simulink model "Robot_Sim_bkp"  (R2017a)
settings: Solver=VariableStepAuto  StartTime=0.0  StopTime=Tsim  FixedStep=Ts_compute  RelTol=1e-3
values from neighbouring files (symbols this model uses):
  A = [0 ur2 0;-ur2 0 ur1;0 0 0]    [Model_old.m]    (also in PIController.m)
  b = 0.1    [Model_old.m]
  C = eye(3)    [Model_old.m]    (also in PIController.m)
  g = 40    [Model_old.m]    (also in ModeloBase_OLD.m)
  Gyro_bias = 0.004    [Model_old.m]
  Kd = 0    [Model_old.m]
  Ki = 10.0    (= 10)    [Model_old.m]
  Kp = 5.0    (= 5)    [Model_old.m]
  ksi = 0.6    [Model_old.m]    (also in ModeloBase_OLD.m = 0.3)
  Rv = var(noise.data)    [Model_old.m]
  Ts = 0.1    [Model_old.m]    (also in ModeloBase_OLD.m; PIController.m)
  Ts_sensor = 1/50    (= 0.02)    [Model_old.m]
undefined symbols (not defined in the file or in its folder): DiscIntNeverNeededParam, K_LQ, Rn, Rw, Ts_compute, Vd
libraries: simulink x27, cstblocks x11
settings Model: PauseTimes=28  NumberOfSteps=10  Creator=davi2  LastModifiedBy=marcus

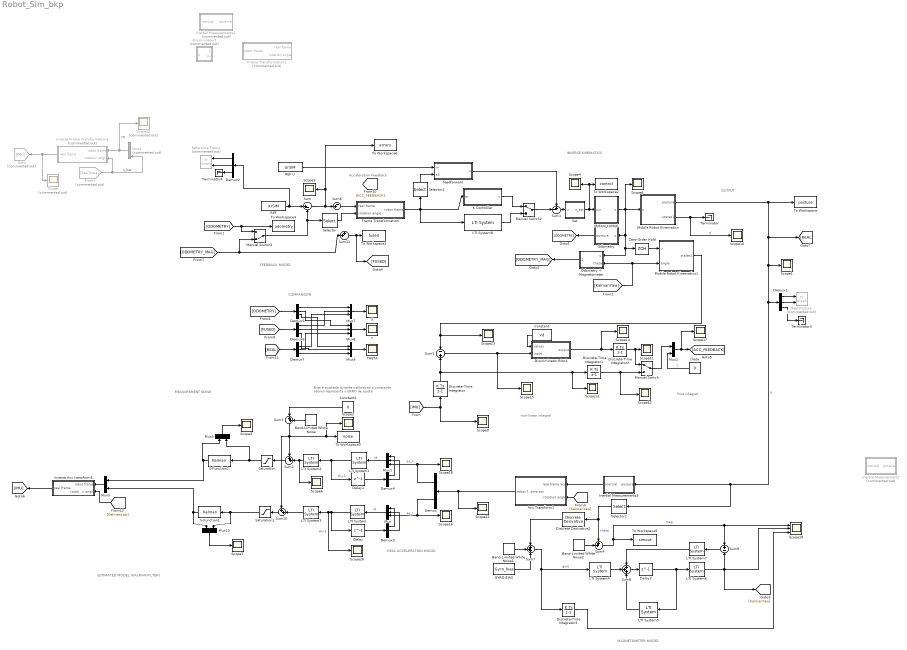
== system Robot_Sim_bkp ==
  note: COMPARISON
  note: Bias é ajustada durante calibracao
      | a constante abaixo representa o ERRO de ajuste
  note: Pure integral
  note: Acceleration Feedback
  note: OUTPUT
  note: MEASUREMENT NOISE
  note: REAL ACCELERATION
      | MODEL
  note: INVERSE KINEMATICS
  note: MAGNETOMETER MODEL
  note: FEEDBACK MODEL
  note: ESTIMATED MODEL (KALMAN FILTER)
  note: non-linear integral
  Acc Transform1 : Subsystem
  Band-Limited White Noise : simulink/Sources/Band-Limited White Noise  Cov=0.0001  Ts=Ts_sensor  seed=[23341]
  Band-Limited White Noise1 : simulink/Sources/Band-Limited White Noise  Cov=0.00001  Ts=Ts_sensor  seed=[23341]
  Band-Limited White Noise2 : simulink/Sources/Band-Limited White Noise  Cov=Rn^2  Ts=Ts_sensor  seed=[23341]
  Constant : Constant  Value=Vd
  Constant2 : Constant  Value=0
  Delay : Delay  DelayLength=1
  Delay1 : Delay  DelayLength=1
  Delay2 : Delay  DelayLength=1
  Demux : Demux  Outputs=2
  Demux{1..7} (7 alike) : Demux  Outputs=3
  Discrete Derivative2 : simulink/Discrete/Discrete Derivative  gainval=1.0  ICPrevScaledInput=0.0  OutMin=[]  OutMax=[]  OutDataType=fixdt(1, 16)  OutScaling=2^-10  DoSatur=off
  Discrete-Time Integrator : DiscreteIntegrator  InitialConditionSetting=State (most efficient)  SampleTime=-1  ICPrevOutput=DiscIntNeverNeededParam  ICPrevScaledInput=DiscIntNeverNeededParam
  Discrete-Time Integrator1 : DiscreteIntegrator  InitialConditionSetting=State (most efficient)  SampleTime=Ts_sensor  ICPrevOutput=DiscIntNeverNeededParam  ICPrevScaledInput=DiscIntNeverNeededParam
  Discrete-Time Integrator2 : DiscreteIntegrator  InitialConditionSetting=State (most efficient)  SampleTime=Ts_sensor  ICPrevOutput=DiscIntNeverNeededParam  ICPrevScaledInput=DiscIntNeverNeededParam
  Discrete-Time Integrator3 : DiscreteIntegrator  InitialConditionSetting=State (most efficient)  SampleTime=-1  ICPrevOutput=DiscIntNeverNeededParam  ICPrevScaledInput=DiscIntNeverNeededParam
  Discriminator Block : Subsystem
  Frame Transformation : Subsystem
  Frame Transformation1 : Subsystem  Commented=on
  From5 : From  Commented=on  GotoTag=RealTheta
  GYRO BIAS : Constant  Value=Gyro_bias
  Goto : Goto  Commented=on  GotoTag=IMU
  Inertial Measurements : Subsystem  Commented=on
  Inertial Measurements1 : Subsystem  Commented=on
  Inertial Measurements3 : Subsystem
  Inverse Acc transform1 : Subsystem
  Inverse Frame Transformation1 : Subsystem  Commented=on
  K Controller : Subsystem
  LTI System : cstblocks/LTI System  sys=A  IC=[]
  LTI System1 : cstblocks/LTI System  sys=A  IC=[]
  LTI System2 : cstblocks/LTI System  sys=C  IC=[]
  LTI System3 : cstblocks/LTI System  sys=C  IC=[]
  LTI System4 : cstblocks/LTI System  sys=Bs  IC=[]
  LTI System5 : cstblocks/LTI System  sys=As  IC=[]
  LTI System6 : cstblocks/LTI System  sys=Cs  IC=[]
  LTI System7 : cstblocks/LTI System  sys=K_KALM  IC=[]
  LTI System8 : cstblocks/LTI System  sys=-K_LQ  IC=[]
  Manual Switch : ManualSwitch
  Manual Switch1 : ManualSwitch  CurrentSetting=0
  Manual Switch2 : ManualSwitch
  Mobile Robot Kinematics : Subsystem
  Mobile Robot Kinematics1 : Subsystem
  Motors control : Subsystem
  Mux{,1,7..9} (5 alike) : Mux  Inputs=3
  Mux{2..3,5,10} (4 alike) : Mux  Inputs=2
  Mux4 : Mux  Commented=on  Inputs=3
  Odometry : Subsystem
  Odometry + Magnetometer : Subsystem
  REF : FromWorkspace  VariableName=XrSIM  SampleTime=Ts  OutputAfterFinalValue=Holding final value
  REF U : FromWorkspace  VariableName=UrSIM  SampleTime=Ts  OutputAfterFinalValue=Holding final value
  Real Posture : simulink/Sinks/XY Graph  Commented=on  xmin=0  xmax=3  ymin=-0.8  ymax=1.5  st=Ts
  Reference Frame : simulink/Sinks/XY Graph  Commented=on  xmin=0  xmax=2  ymin=0  ymax=1.5  st=Ts
  S-Function1 : S-Function  FunctionName=Kalman  Parameters=Ts_sensor,A,C,Rw,Rv  SFunctionDeploymentMode=off  EnableBusSupport=off  mask{Ts=Ts_sensor, A=A, C=C, Rv=Rv, Rw=Rw}
      mask prompts: Ts "Tempo de Amostragem"; A "Matriz A"; C "Matriz C"; Rv "Covariancia da Saida"; Rw "Covariancia do Processo"
      mask DialogControl DescTextVar Tooltip: Filtro
      mask Display: disp('MyKalman')
  S-Function2 : S-Function  FunctionName=Kalman  Parameters=Ts_sensor,A,C,Rw,Rv  SFunctionDeploymentMode=off  EnableBusSupport=off  mask{Ts=Ts_sensor, A=A, C=C, Rv=Rv, Rw=Rw}
      mask prompts: Ts "Tempo de Amostragem"; A "Matriz A"; C "Matriz C"; Rv "Covariancia da Saida"; Rw "Covariancia do Processo"
      mask DialogControl DescTextVar Tooltip: Filtro
      mask Display: disp('MyKalman')
  Sat : Subsystem
  Saturation : Saturate  UpperLimit=4*9.8  LowerLimit=-4*9.8
  Saturation1 : Saturate  UpperLimit=4*9.8  LowerLimit=-4*9.8
  Scope : Scope  Commented=on
  Scope{1..18,22..23,26} (21 alike) : Scope
  Scope19 : Scope  NumInputPorts=3
  Scope21 : Scope  Commented=on
  Selector : Selector  InputPortWidth=3  IndexOptions=Index vector (dialog)  Indices=3  OutputSizes=1
  Selector1 : Selector  InputPortWidth=3  IndexOptions=Index vector (dialog)  Indices=3  OutputSizes=1
  Selector2 : Selector  InputPortWidth=3  IndexOptions=Index vector (dialog)  Indices=3  OutputSizes=1
  Sum : Sum  Inputs=|+-
  Sum1 : Sum  Inputs=+-|
  Sum{2,4,10..11} (4 alike) : Sum  Inputs=++|
  Sum3 : Sum  Inputs=|++
  Sum5 : Sum  Inputs=-+
  Sum6 : Sum  Inputs=-+|
  Sum7 : Sum  Inputs=+++
  Sum8 : Sum  Inputs=+++
  Sum9 : Sum  Inputs=+-
  THETA : Scope
  Terminator : Terminator
  Terminator3 : Terminator
  Terminator4 : Terminator
  To Workspace : ToWorkspace  VariableName=posture  SaveFormat=Timeseries  SampleTime=-1
  To Workspace1 : ToWorkspace  VariableName=fused  SaveFormat=Timeseries  SampleTime=-1
  To Workspace2 : ToWorkspace  VariableName=control  SaveFormat=Timeseries  SampleTime=-1
  To Workspace3 : ToWorkspace  VariableName=noise  SaveFormat=Timeseries  SampleTime=-1
  To Workspace4 : ToWorkspace  VariableName=odometry  SaveFormat=Timeseries  SampleTime=-1
  To Workspace5 : ToWorkspace  VariableName=simout  SaveFormat=Timeseries  SampleTime=-1
  To Workspace6 : ToWorkspace  VariableName=errors  SaveFormat=Timeseries  SampleTime=-1
  X : Scope
  Y : Scope
  Zero-Order Hold : ZeroOrderHold  SampleTime=-1
  discriminator5 : Subsystem  Commented=on
  feedforward : Subsystem
  theta : Constant  Value=0
  wires:
  Frame Transformation/1(robot frame) -> LTI System8/1, K Controller/1(er), Selector1/1
  REF U/1 -> feedforward/1(ur)
  Selector1/1 -> feedforward/2(e3)
  Motors control/1(u) -> Odometry + Magnetometer/1(u), Zero-Order Hold/1, Odometry/1(u), Mobile Robot Kinematics/1(u), Scope8/1
  Selector2/1 -> Sum4/1, Discrete Derivative2/1  "theta"
  Demux1/1 -> Real Posture/1
  Demux1/2 -> Real Posture/2
  REF/1 -> Demux2/1, Sum/1
  Odometry/1(posture) -> [ODOMETRY]
  Sum1/1 -> Sat/1(u)
  Sat/1(u_sat) -> Motors control/1(uin), Scope4/1, To Workspace2/1
  Demux1/3 -> Terminator3/1
  Band-Limited White Noise2/1 -> Sum4/2
  Demux2/1 -> Reference Frame/1
  Demux2/2 -> Reference Frame/2
  Demux2/3 -> Terminator4/1
  LTI System/1 -> Scope26/1, LTI System3/1, Delay/1  "xk+1"
  Delay/1 -> Demux3/1
  Demux3/1 -> Mux/1
  Demux3/2 -> Mux/2
  Mux/1 -> LTI System/1  "xk"
  Demux4/2 -> Mux1/2
  Delay1/1 -> Demux4/1
  Demux4/1 -> Mux1/1
  LTI System1/1 -> Delay1/1, LTI System2/1  "xk+1"
  Mux1/1 -> LTI System1/1  "xk"
  Inverse Frame Transformation1/1(real frame) -> Goto/1, Scope/1
  From5/1 -> Mux4/3, Inverse Frame Transformation1/2(rotation angle)  "t_hat"
  LTI System3/1 -> Sum10/2
  Mux4/1 -> Scope21/1, Inverse Frame Transformation1/1(robot frame)  "im"
  Mobile Robot Kinematics/1(posture) -> [REAL], Selector2/1, Inertial Measurements3/1(posture), Demux1/1, Scope1/1, To Workspace/1  "P"
  Demux/1 -> Mux1/3, Scope18/1  "ax_r"
  Demux/2 -> Scope16/1, Mux/3  "ay_r"
  Inertial Measurements3/1(inercial) -> Acc Transform1/1(real frame acc)
  Acc Transform1/1(robot frame acc) -> Scope22/1, Demux/1
  Sum6/1 -> Frame Transformation/1(real frame)
  theta/1 -> Mux2/2  "t"
  Mux2/1 -> Scope17/1, [ACC_FEEDBACK]
  LTI System2/1 -> Scope6/1, Sum2/2
  Sum11/1 -> [FUSED], To Workspace1/1
  Mux5/1 -> Scope5/1
  Discrete-Time Integrator2/1 -> Scope11/1, Manual Switch/1
  Discrete-Time Integrator1/1 -> Manual Switch/2, Scope12/1
  Manual Switch/1 -> Mux2/1
  Discriminator Block/1(output) -> Discrete-Time Integrator2/1, Scope14/1
  Selector/1 -> Frame Transformation/2(rotation angle)
  [KalmanYaw] -> Acc Transform1/2(rotation angle)
  Odometry + Magnetometer/1(posture) -> [ODOMETRY_MAG]
  [KalmanYaw] -> Odometry + Magnetometer/2(theta), Mobile Robot Kinematics1/2(angle)
  [ODOMETRY] -> Manual Switch1/1, To Workspace4/1
  [ODOMETRY_MAG] -> Sum11/2, Manual Switch1/2
  Manual Switch1/1 -> Selector/1, Sum/2
  [ODOMETRY] -> Demux5/1
  [FUSED] -> Demux6/1
  [REAL] -> Demux7/1
  Demux5/1 -> Mux7/1
  Demux6/1 -> Mux7/2
  Demux7/1 -> Mux7/3
  Mux7/1 -> X/1
  Demux5/2 -> Mux8/1
  Demux6/2 -> Mux8/2
  Demux7/2 -> Mux8/3
  Demux5/3 -> Mux9/1
  Demux6/3 -> Mux9/2
  Demux7/3 -> Mux9/3
  Mux8/1 -> Y/1
  Mux9/1 -> THETA/1
  Mobile Robot Kinematics/2(states1) -> Scope10/1, Terminator/1  "p'"
  Mux3/1 -> Inverse Acc transform1/1(robot frame)
  [KalmanYaw] -> Inverse Acc transform1/2(rotation angle)
  Inverse Acc transform1/1(real frame) -> [IMU]
  Constant/1 -> Discriminator Block/1(values)
  Sum3/1 -> Sum10/1, Sum2/1, Scope2/1, To Workspace3/1
  Band-Limited White Noise/1 -> Sum3/2
  Constant2/1 -> Sum3/1
  Sum10/1 -> Saturation1/1
  Sum2/1 -> Saturation/1
  Saturation1/1 -> S-Function1/1, Mux10/2
  Saturation/1 -> S-Function2/1, Mux5/2
  Mux10/1 -> Scope7/1
  Zero-Order Hold/1 -> Mobile Robot Kinematics1/1(u)
  [IMU] -> Discrete-Time Integrator/1, Scope9/1
  Sum5/1 -> Scope15/1, Discriminator Block/2(input)
  Discrete-Time Integrator/1 -> Scope13/1, Discrete-Time Integrator1/1, Sum5/2
  S-Function1/1 -> Mux3/2, Mux10/1
  Mobile Robot Kinematics1/1(states1) -> Scope23/1, Sum5/1
  S-Function2/1 -> Mux3/1, Mux5/1
  Band-Limited White Noise1/1 -> Sum7/2
  Discrete Derivative2/1 -> Sum7/1
  GYRO BIAS/1 -> Sum7/3
  Sum7/1 -> Discrete-Time Integrator3/1, LTI System4/1  "gyro"
  Sum4/1 -> To Workspace5/1, Scope19/1, Sum9/1  "mag"
  Sum8/1 -> Delay2/1
  LTI System4/1 -> Sum8/2
  Delay2/1 -> LTI System6/1, LTI System5/1
  LTI System5/1 -> Sum8/3
  LTI System7/1 -> Sum8/1
  LTI System6/1 -> Scope19/2, [KalmanYaw], Sum9/2
  Sum9/1 -> LTI System7/1
  Discrete-Time Integrator3/1 -> Scope19/3
  Sum/1 -> Sum6/2, To Workspace6/1, Scope3/1
  Manual Switch2/1 -> Sum1/2
  feedforward/1(u) -> Sum1/1
  LTI System8/1 -> Manual Switch2/2
  K Controller/1(v) -> Manual Switch2/1

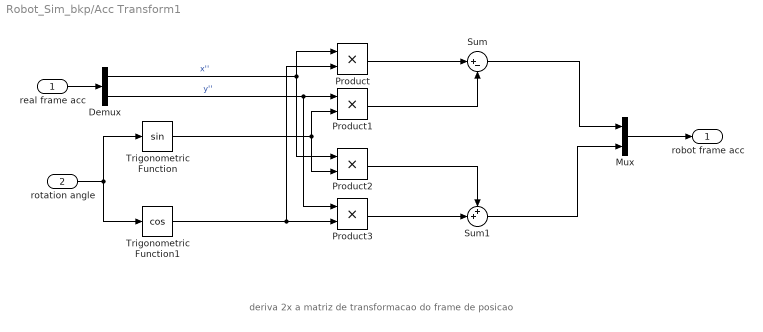
== system Robot_Sim_bkp/Acc Transform1 ==
  note: deriva 2x a matriz de transformacao do frame de posicao
  real frame acc : Inport
  rotation angle : Inport  Port=2
  Demux : Demux  Outputs=2
  Mux : Mux  Inputs=2
  Product{,1..3} (4 alike) : Product
  Sum : Sum  Inputs=|+-
  Sum1 : Sum  Inputs=++|
  Trigonometric Function : Trigonometry
  Trigonometric Function1 : Trigonometry  Operator=cos
  robot frame acc : Outport
  wires:
  rotation angle/1 -> Trigonometric Function/1, Trigonometric Function1/1
  Mux/1 -> robot frame acc/1
  real frame acc/1 -> Demux/1
  Demux/1 -> Product2/1, Product/1  "x''"
  Trigonometric Function1/1 -> Product/2, Product3/2
  Product/1 -> Sum/1
  Trigonometric Function/1 -> Product1/2, Product2/2
  Demux/2 -> Product3/1, Product1/1  "y''"
  Product1/1 -> Sum/2
  Sum/1 -> Mux/1
  Product3/1 -> Sum1/2
  Product2/1 -> Sum1/1
  Sum1/1 -> Mux/2

== system Robot_Sim_bkp/Discriminator Block ==
  values : Inport
  input : Inport  Port=2
  Demux : Demux  Outputs=2
  Mux : Mux  Inputs=2
  discriminator1 : Subsystem
  discriminator3 : Subsystem
  output : Outport
  wires:
  input/1 -> Demux/1
  Demux/1 -> discriminator3/2(IN)
  Demux/2 -> discriminator1/2(IN)
  Mux/1 -> output/1
  discriminator3/1(OUT) -> Mux/1
  discriminator1/1(OUT) -> Mux/2
  values/1 -> discriminator1/1(value), discriminator3/1(value)

== system Robot_Sim_bkp/Frame Transformation ==
  real frame : Inport
  rotation angle : Inport  Port=2
  Mux : Mux  Inputs=2
  S-Function : S-Function  FunctionName=Real2Robot  Parameters=Ts  SFunctionDeploymentMode=off  EnableBusSupport=off
  robot frame : Outport
  wires:
  real frame/1 -> Mux/1
  rotation angle/1 -> Mux/2
  Mux/1 -> S-Function/1
  S-Function/1 -> robot frame/1

== system Robot_Sim_bkp/Frame Transformation1 ==
  real frame : Inport
  rotation angle : Inport  Port=2
  Mux : Mux  Inputs=2
  S-Function : S-Function  FunctionName=Real2Robot  Parameters=Ts_compute  SFunctionDeploymentMode=off  EnableBusSupport=off
  robot frame : Outport
  wires:
  real frame/1 -> Mux/1
  rotation angle/1 -> Mux/2
  Mux/1 -> S-Function/1
  S-Function/1 -> robot frame/1

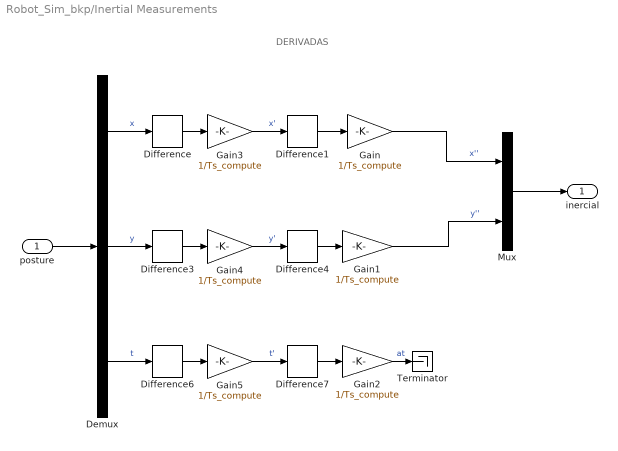
== system Robot_Sim_bkp/Inertial Measurements ==
  note: DERIVADAS
  posture : Inport
  Demux : Demux  Outputs=3
  Difference{,1,3..4,6..7} (6 alike) : simulink/Discrete/Difference  ICPrevInput=0.0  OutMin=[]  OutMax=[]  OutDataType=fixdt(1, 16)  OutScaling=2^-10  DoSatur=off
  Gain{,1..5} (6 alike) : Gain  Gain=1/Ts_compute
  Mux : Mux  Inputs=2
  Terminator : Terminator
  inercial : Outport
  wires:
  posture/1 -> Demux/1
  Demux/3 -> Difference6/1  "t"
  Demux/2 -> Difference3/1  "y"
  Demux/1 -> Difference/1  "x"
  Difference1/1 -> Gain/1
  Difference4/1 -> Gain1/1
  Difference7/1 -> Gain2/1
  Mux/1 -> inercial/1
  Gain2/1 -> Terminator/1  "at"
  Difference/1 -> Gain3/1
  Gain3/1 -> Difference1/1  "x'"
  Difference3/1 -> Gain4/1
  Gain4/1 -> Difference4/1  "y'"
  Difference6/1 -> Gain5/1
  Gain5/1 -> Difference7/1  "t'"
  Gain/1 -> Mux/1  "x''"
  Gain1/1 -> Mux/2  "y''"

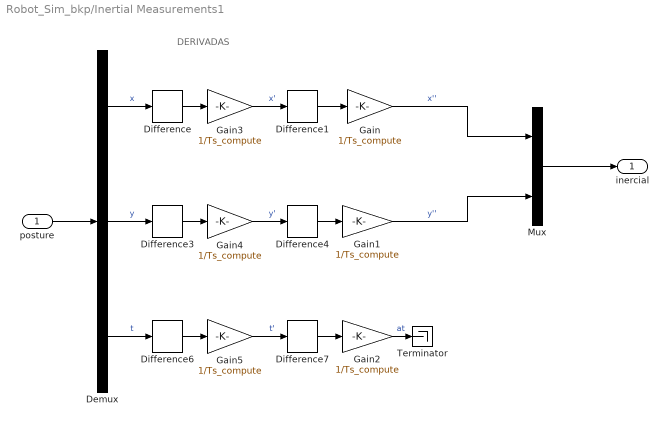
== system Robot_Sim_bkp/Inertial Measurements1 ==
  note: DERIVADAS
  posture : Inport
  Demux : Demux  Outputs=3
  Difference{,1,3..4,6..7} (6 alike) : simulink/Discrete/Difference  ICPrevInput=0.0  OutMin=[]  OutMax=[]  OutDataType=fixdt(1, 16)  OutScaling=2^-10  DoSatur=off
  Gain{,1..5} (6 alike) : Gain  Gain=1/Ts_compute
  Mux : Mux  Inputs=2
  Terminator : Terminator
  inercial : Outport
  wires:
  posture/1 -> Demux/1
  Demux/3 -> Difference6/1  "t"
  Demux/2 -> Difference3/1  "y"
  Demux/1 -> Difference/1  "x"
  Difference1/1 -> Gain/1
  Difference4/1 -> Gain1/1
  Difference7/1 -> Gain2/1
  Mux/1 -> inercial/1
  Gain2/1 -> Terminator/1  "at"
  Difference/1 -> Gain3/1
  Gain3/1 -> Difference1/1  "x'"
  Difference3/1 -> Gain4/1
  Gain4/1 -> Difference4/1  "y'"
  Difference6/1 -> Gain5/1
  Gain5/1 -> Difference7/1  "t'"
  Gain/1 -> Mux/1  "x''"
  Gain1/1 -> Mux/2  "y''"

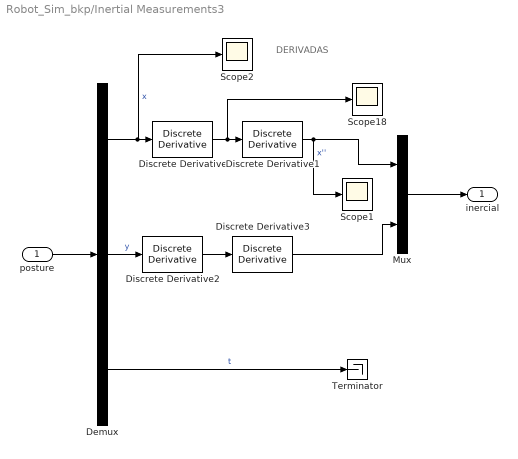
== system Robot_Sim_bkp/Inertial Measurements3 ==
  note: DERIVADAS
  posture : Inport
  Demux : Demux  Outputs=3
  Discrete Derivative{,1..3} (4 alike) : simulink/Discrete/Discrete Derivative  gainval=1.0  ICPrevScaledInput=0.0  OutMin=[]  OutMax=[]  OutDataType=fixdt(1, 16)  OutScaling=2^-10  DoSatur=off
  Mux : Mux  Inputs=2
  Scope1 : Scope
  Scope18 : Scope
  Scope2 : Scope
  Terminator : Terminator
  inercial : Outport
  wires:
  posture/1 -> Demux/1
  Demux/1 -> Discrete Derivative/1, Scope2/1  "x"
  Mux/1 -> inercial/1
  Discrete Derivative1/1 -> Scope1/1, Mux/1  "x''"
  Discrete Derivative/1 -> Scope18/1, Discrete Derivative1/1
  Demux/2 -> Discrete Derivative2/1  "y"
  Discrete Derivative2/1 -> Discrete Derivative3/1
  Discrete Derivative3/1 -> Mux/2
  Demux/3 -> Terminator/1  "t"

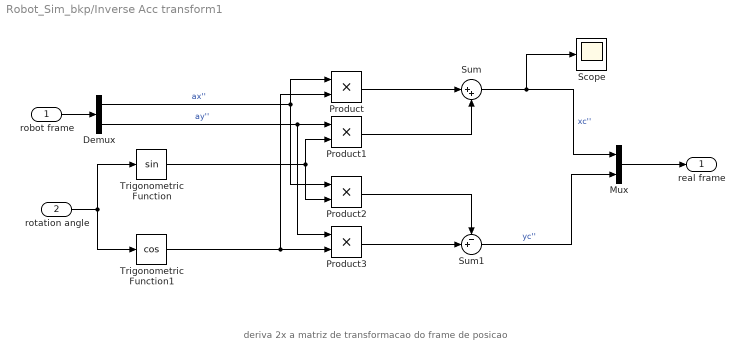
== system Robot_Sim_bkp/Inverse Acc transform1 ==
  note: deriva 2x a matriz de transformacao do frame de posicao
  robot frame : Inport
  rotation angle : Inport  Port=2
  Demux : Demux  Outputs=2
  Mux : Mux  Inputs=2
  Product{,1..3} (4 alike) : Product
  Scope : Scope
  Sum : Sum  Inputs=|++
  Sum1 : Sum  Inputs=-+|
  Trigonometric Function : Trigonometry
  Trigonometric Function1 : Trigonometry  Operator=cos
  real frame : Outport
  wires:
  rotation angle/1 -> Trigonometric Function/1, Trigonometric Function1/1
  Mux/1 -> real frame/1
  robot frame/1 -> Demux/1
  Demux/1 -> Product2/1, Product/1  "ax''"
  Trigonometric Function1/1 -> Product/2, Product3/2
  Product/1 -> Sum/1
  Trigonometric Function/1 -> Product1/2, Product2/2
  Demux/2 -> Product3/1, Product1/1  "ay''"
  Product1/1 -> Sum/2
  Sum/1 -> Scope/1, Mux/1  "xc''"
  Product3/1 -> Sum1/2
  Product2/1 -> Sum1/1
  Sum1/1 -> Mux/2  "yc''"

== system Robot_Sim_bkp/Inverse Frame Transformation1 ==
  robot frame : Inport
  rotation angle : Inport  Port=2
  Mux : Mux  Inputs=2
  S-Function : S-Function  FunctionName=Robot2Real  Parameters=Ts  SFunctionDeploymentMode=off  EnableBusSupport=off
  real frame : Outport
  wires:
  S-Function/1 -> real frame/1
  Mux/1 -> S-Function/1
  rotation angle/1 -> Mux/2
  robot frame/1 -> Mux/1

== system Robot_Sim_bkp/K Controller ==
  er : Inport
  Constant : Constant  Value=ksi
  Constant1 : Constant  Value=g
  Mux : Mux  Inputs=5
  S-Function : S-Function  FunctionName=ControllerK  Parameters=Ts  SFunctionDeploymentMode=off  EnableBusSupport=off
  v : Outport
  wires:
  er/1 -> Mux/1
  [vr] -> Mux/2
  [wr] -> Mux/3
  Constant/1 -> Mux/4
  Constant1/1 -> Mux/5
  Mux/1 -> S-Function/1
  S-Function/1 -> v/1

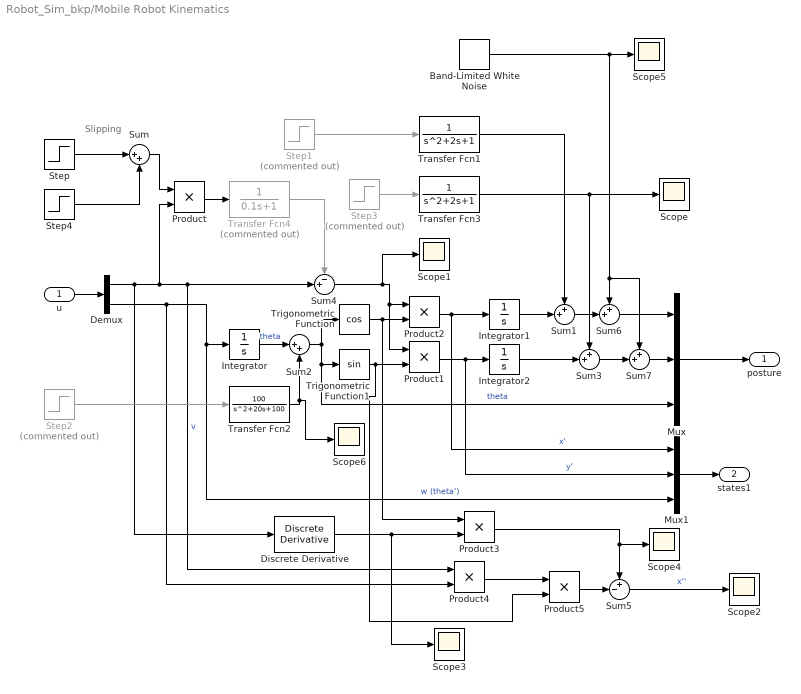
== system Robot_Sim_bkp/Mobile Robot Kinematics ==
  note: Slipping
  u : Inport
  Band-Limited White Noise : simulink/Sources/Band-Limited White Noise  Cov=0  Ts=0.05  seed=[23341]
  Demux : Demux  Outputs=2
  Discrete Derivative : simulink/Discrete/Discrete Derivative  gainval=1.0  ICPrevScaledInput=0.0  OutMin=[]  OutMax=[]  OutDataType=fixdt(1, 16)  OutScaling=2^-10  DoSatur=off
  Integrator : Integrator
  Integrator1 : Integrator
  Integrator2 : Integrator
  Mux : Mux  Inputs=3
  Mux1 : Mux  Inputs=3
  Product{,1..5} (6 alike) : Product
  Scope{,1..6} (7 alike) : Scope
  Step : Step  Time=25  SampleTime=0
  Step1 : Step  Commented=on  Time=20  After=0.7  SampleTime=0
  Step2 : Step  Commented=on  Time=10  After=0.5  SampleTime=0
  Step3 : Step  Commented=on  Time=5  After=-0.7  SampleTime=0
  Step4 : Step  Time=27  After=-1  SampleTime=0
  Sum : Sum  Inputs=|++
  Sum{1,3,6..7} (4 alike) : Sum  Inputs=++|
  Sum2 : Sum  Inputs=|++
  Sum4 : Sum  Inputs=-+|
  Sum5 : Sum  Inputs=+-|
  Transfer Fcn1 : TransferFcn  Numerator=1
  Transfer Fcn2 : TransferFcn  Numerator=100  Denominator=[1 20 100]
  Transfer Fcn3 : TransferFcn  Numerator=1
  Transfer Fcn4 : TransferFcn  Commented=on  Numerator=1  Denominator=[0.1 1]
  Trigonometric Function : Trigonometry  Operator=cos
  Trigonometric Function1 : Trigonometry
  posture : Outport
  states1 : Outport  Port=2
  wires:
  u/1 -> Demux/1
  Demux/2 -> Product4/2, Integrator/1, Mux1/3  "w (theta')"
  Trigonometric Function/1 -> Product3/1, Product2/2
  Demux/1 -> Discrete Derivative/1, Product4/1, Sum4/2, Product/2  "v"
  Trigonometric Function1/1 -> Product5/2, Product1/2
  Mux/1 -> posture/1
  Step2/1 -> Transfer Fcn2/1
  Integrator/1 -> Sum2/1  "theta"
  Sum2/1 -> Mux/3, Trigonometric Function1/1, Trigonometric Function/1  "theta"
  Transfer Fcn2/1 -> Scope6/1, Sum2/2
  Product1/1 -> Mux1/2, Integrator2/1  "y'"
  Product2/1 -> Mux1/1, Integrator1/1  "x'"
  Step1/1 -> Transfer Fcn1/1
  Step3/1 -> Transfer Fcn3/1
  Integrator1/1 -> Sum1/2
  Integrator2/1 -> Sum3/2
  Transfer Fcn3/1 -> Sum3/1, Scope/1
  Transfer Fcn1/1 -> Sum1/1
  Step/1 -> Sum/1
  Step4/1 -> Sum/2
  Sum/1 -> Product/1
  Sum4/1 -> Scope1/1, Product1/1, Product2/1
  Product/1 -> Transfer Fcn4/1
  Transfer Fcn4/1 -> Sum4/1
  Mux1/1 -> states1/1
  Discrete Derivative/1 -> Scope3/1, Product3/2
  Product3/1 -> Scope4/1, Sum5/1
  Sum5/1 -> Scope2/1  "x''"
  Product4/1 -> Product5/1
  Product5/1 -> Sum5/2
  Sum1/1 -> Sum6/2
  Sum3/1 -> Sum7/2
  Sum7/1 -> Mux/2
  Sum6/1 -> Mux/1
  Band-Limited White Noise/1 -> Scope5/1, Sum7/1, Sum6/1

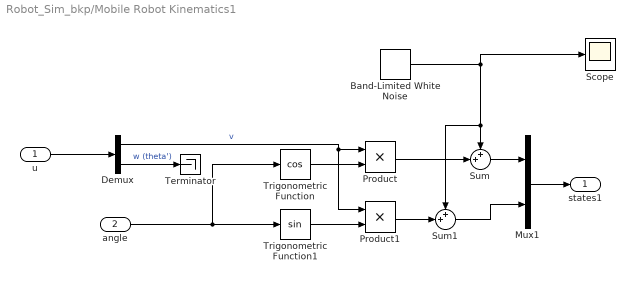
== system Robot_Sim_bkp/Mobile Robot Kinematics1 ==
  u : Inport
  angle : Inport  Port=2
  Band-Limited White Noise : simulink/Sources/Band-Limited White Noise  Cov=0.05^4  Ts=0.1  seed=[23341]
  Demux : Demux  Outputs=2
  Mux1 : Mux  Inputs=2
  Product : Product
  Product1 : Product
  Scope : Scope
  Sum : Sum  Inputs=++|
  Sum1 : Sum  Inputs=++|
  Terminator : Terminator
  Trigonometric Function : Trigonometry  Operator=cos
  Trigonometric Function1 : Trigonometry
  states1 : Outport
  wires:
  u/1 -> Demux/1
  Demux/1 -> Product1/1, Product/1  "v"
  Mux1/1 -> states1/1
  Trigonometric Function/1 -> Product/2
  Trigonometric Function1/1 -> Product1/2
  Product/1 -> Sum/2
  Product1/1 -> Sum1/2
  Band-Limited White Noise/1 -> Scope/1, Sum1/1, Sum/1
  Sum/1 -> Mux1/1
  Sum1/1 -> Mux1/2
  angle/1 -> Trigonometric Function/1, Trigonometric Function1/1
  Demux/2 -> Terminator/1  "w (theta')"

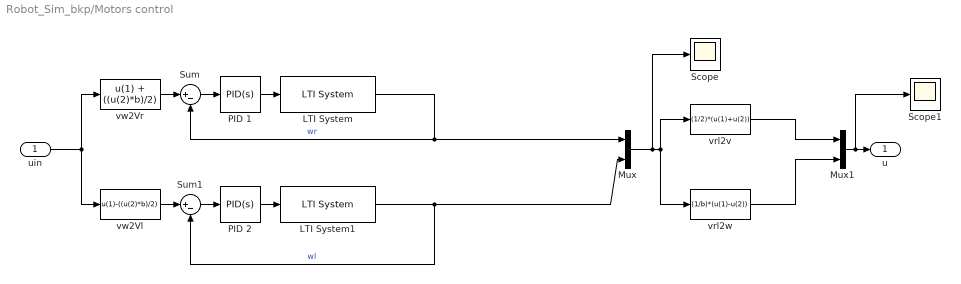
== system Robot_Sim_bkp/Motors control ==
  uin : Inport
  LTI System : cstblocks/LTI System  sys=HMotor  IC=[]
  LTI System1 : cstblocks/LTI System  sys=HMotor  IC=[]
  Mux : Mux  Inputs=2
  Mux1 : Mux  Inputs=2
  PID 1 : simulink/Continuous/PID Controller  Controller=PID  TimeDomain=Continuous-time  SampleTime=-1  IntegratorMethod=Forward Euler  FilterMethod=Forward Euler  Form=Parallel  UseFilter=on  ControllerParametersSource=internal  P=Kp  I=Ki  D=Kd  N=100  InitialConditionSource=internal  InitialConditionForIntegrator=0  InitialConditionForFilter=0  ExternalReset=none  LimitOutput=off  UpperSaturationLimit=inf  LowerSaturationLimit=-inf  LinearizeAsGain=on  AntiWindupMode=none  Kb=1  TrackingMode=off  Kt=1  PParamMin=[]  PParamMax=[]  IParamMin=[]  IParamMax=[]  DParamMin=[]  DParamMax=[]  NParamMin=[]  NParamMax=[]  KbParamMin=[]  KbParamMax=[]  KtParamMin=[]  KtParamMax=[]  POutMin=[]  POutMax=[]  IOutMin=[]  IOutMax=[]  DOutMin=[]  DOutMax=[]  NOutMin=[]  NOutMax=[]  KbOutMin=[]  KbOutMax=[]  KtOutMin=[]  KtOutMax=[]  IntegratorOutMin=[]  IntegratorOutMax=[]  FilterOutMin=[]  FilterOutMax=[]  SumOutMin=[]  SumOutMax=[]  SumI1OutMin=[]  SumI1OutMax=[]  SumI2OutMin=[]  SumI2OutMax=[]  SumI3OutMin=[]  SumI3OutMax=[]  SumDOutMin=[]  SumDOutMax=[]  SaturationOutMin=[]  SaturationOutMax=[]  IntegratorContinuousStateAttributes=''  IntegratorStateMustResolveToSignalObject=off  IntegratorRTWStateStorageClass=Auto  FilterContinuousStateAttributes=''  FilterStateMustResolveToSignalObject=off  FilterRTWStateStorageClass=Auto  DifferentiatorICPrevScaledInput=0  DifferentiatorOutMin=[]  DifferentiatorOutMax=[]  InitialConditionSetting=State (most efficient)
  PID 2 : simulink/Continuous/PID Controller  Controller=PID  TimeDomain=Continuous-time  SampleTime=-1  IntegratorMethod=Forward Euler  FilterMethod=Forward Euler  Form=Parallel  UseFilter=on  ControllerParametersSource=internal  P=Kp  I=Ki  D=Kd  N=100  InitialConditionSource=internal  InitialConditionForIntegrator=0  InitialConditionForFilter=0  ExternalReset=none  LimitOutput=off  UpperSaturationLimit=inf  LowerSaturationLimit=-inf  LinearizeAsGain=on  AntiWindupMode=none  Kb=1  TrackingMode=off  Kt=1  PParamMin=[]  PParamMax=[]  IParamMin=[]  IParamMax=[]  DParamMin=[]  DParamMax=[]  NParamMin=[]  NParamMax=[]  KbParamMin=[]  KbParamMax=[]  KtParamMin=[]  KtParamMax=[]  POutMin=[]  POutMax=[]  IOutMin=[]  IOutMax=[]  DOutMin=[]  DOutMax=[]  NOutMin=[]  NOutMax=[]  KbOutMin=[]  KbOutMax=[]  KtOutMin=[]  KtOutMax=[]  IntegratorOutMin=[]  IntegratorOutMax=[]  FilterOutMin=[]  FilterOutMax=[]  SumOutMin=[]  SumOutMax=[]  SumI1OutMin=[]  SumI1OutMax=[]  SumI2OutMin=[]  SumI2OutMax=[]  SumI3OutMin=[]  SumI3OutMax=[]  SumDOutMin=[]  SumDOutMax=[]  SaturationOutMin=[]  SaturationOutMax=[]  IntegratorContinuousStateAttributes=''  IntegratorStateMustResolveToSignalObject=off  IntegratorRTWStateStorageClass=Auto  FilterContinuousStateAttributes=''  FilterStateMustResolveToSignalObject=off  FilterRTWStateStorageClass=Auto  DifferentiatorICPrevScaledInput=0  DifferentiatorOutMin=[]  DifferentiatorOutMax=[]  InitialConditionSetting=State (most efficient)
  Scope : Scope
  Scope1 : Scope
  Sum : Sum  Inputs=|+-
  Sum1 : Sum  Inputs=|+-
  vrl2v : Fcn  Expr=(1/2)*(u(1)+u(2))
  vrl2w : Fcn  Expr=(1/b)*(u(1)-u(2))
  vw2Vl : Fcn  Expr=u(1)-((u(2)*b)/2)
  vw2Vr : Fcn  Expr=u(1) + ((u(2)*b)/2)
  u : Outport
  wires:
  vw2Vr/1 -> Sum/1
  LTI System1/1 -> Mux/2, Sum1/2  "wl"
  vw2Vl/1 -> Sum1/1
  Sum1/1 -> PID 2/1
  PID 2/1 -> LTI System1/1
  Sum/1 -> PID 1/1
  PID 1/1 -> LTI System/1
  LTI System/1 -> Mux/1, Sum/2  "wr"
  uin/1 -> vw2Vl/1, vw2Vr/1
  Mux/1 -> Scope/1, vrl2v/1, vrl2w/1
  Mux1/1 -> Scope1/1, u/1
  vrl2v/1 -> Mux1/1
  vrl2w/1 -> Mux1/2

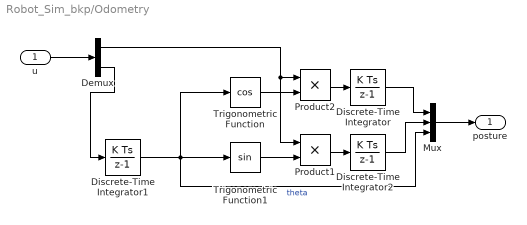
== system Robot_Sim_bkp/Odometry ==
  u : Inport
  Demux : Demux  Outputs=2
  Discrete-Time Integrator : DiscreteIntegrator  InitialConditionSetting=State (most efficient)  SampleTime=Ts  ICPrevOutput=DiscIntNeverNeededParam  ICPrevScaledInput=DiscIntNeverNeededParam
  Discrete-Time Integrator1 : DiscreteIntegrator  InitialConditionSetting=State (most efficient)  SampleTime=Ts  ICPrevOutput=DiscIntNeverNeededParam  ICPrevScaledInput=DiscIntNeverNeededParam
  Discrete-Time Integrator2 : DiscreteIntegrator  InitialConditionSetting=State (most efficient)  SampleTime=Ts  ICPrevOutput=DiscIntNeverNeededParam  ICPrevScaledInput=DiscIntNeverNeededParam
  Mux : Mux  Inputs=3
  Product1 : Product
  Product2 : Product
  Trigonometric Function : Trigonometry  Operator=cos
  Trigonometric Function1 : Trigonometry
  posture : Outport
  wires:
  u/1 -> Demux/1
  Demux/2 -> Discrete-Time Integrator1/1
  Trigonometric Function/1 -> Product2/2
  Demux/1 -> Product1/1, Product2/1
  Product2/1 -> Discrete-Time Integrator/1
  Trigonometric Function1/1 -> Product1/2
  Product1/1 -> Discrete-Time Integrator2/1
  Discrete-Time Integrator/1 -> Mux/1
  Discrete-Time Integrator2/1 -> Mux/2
  Mux/1 -> posture/1
  Discrete-Time Integrator1/1 -> Mux/3, Trigonometric Function1/1, Trigonometric Function/1  "theta"

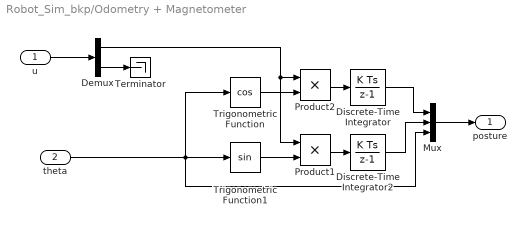
== system Robot_Sim_bkp/Odometry + Magnetometer ==
  u : Inport
  theta : Inport  Port=2
  Demux : Demux  Outputs=2
  Discrete-Time Integrator : DiscreteIntegrator  InitialConditionSetting=State (most efficient)  SampleTime=Ts  ICPrevOutput=DiscIntNeverNeededParam  ICPrevScaledInput=DiscIntNeverNeededParam
  Discrete-Time Integrator2 : DiscreteIntegrator  InitialConditionSetting=State (most efficient)  SampleTime=Ts  ICPrevOutput=DiscIntNeverNeededParam  ICPrevScaledInput=DiscIntNeverNeededParam
  Mux : Mux  Inputs=3
  Product1 : Product
  Product2 : Product
  Terminator : Terminator
  Trigonometric Function : Trigonometry  Operator=cos
  Trigonometric Function1 : Trigonometry
  posture : Outport
  wires:
  u/1 -> Demux/1
  Trigonometric Function/1 -> Product2/2
  Demux/1 -> Product1/1, Product2/1
  Product2/1 -> Discrete-Time Integrator/1
  Trigonometric Function1/1 -> Product1/2
  Product1/1 -> Discrete-Time Integrator2/1
  Discrete-Time Integrator/1 -> Mux/1
  Discrete-Time Integrator2/1 -> Mux/2
  Mux/1 -> posture/1
  Demux/2 -> Terminator/1
  theta/1 -> Mux/3, Trigonometric Function/1, Trigonometric Function1/1

== system Robot_Sim_bkp/Sat ==
  u : Inport
  Demux : Demux  Outputs=2
  Mux : Mux  Inputs=2
  Saturation : Saturate  UpperLimit=0.4  LowerLimit=0
  Saturation1 : Saturate  UpperLimit=0.8  LowerLimit=-0.8
  u_sat : Outport
  wires:
  Demux/2 -> Saturation1/1  "W"
  Demux/1 -> Saturation/1  "V"
  u/1 -> Demux/1
  Saturation/1 -> Mux/1
  Saturation1/1 -> Mux/2
  Mux/1 -> u_sat/1

== system Robot_Sim_bkp/discriminator5 ==
  value : Inport
  IN : Inport  Port=2
  Abs : Abs
  If : If  NumInputs=2  IfExpression=u1 < u2
  If Action Subsystem : Subsystem  TreatAsAtomicUnit=on
  If Action Subsystem1 : Subsystem  TreatAsAtomicUnit=on
  Merge : Merge
  OUT : Outport
  wires:
  IN/1 -> If Action Subsystem1/1(In1), Abs/1
  Abs/1 -> If/1
  If/1 -> If Action Subsystem/Action
  If/2 -> If Action Subsystem1/Action
  If Action Subsystem/1(Out1) -> Merge/1
  If Action Subsystem1/1(Out1) -> Merge/2
  Merge/1 -> OUT/1
  value/1 -> If/2

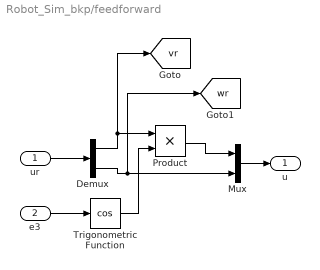
== system Robot_Sim_bkp/feedforward ==
  ur : Inport
  e3 : Inport  Port=2
  Demux : Demux  Outputs=2
  Mux : Mux  Inputs=2
  Product : Product
  Trigonometric Function : Trigonometry  Operator=cos
  u : Outport
  tag scope: vr=global, wr=global
  wires:
  e3/1 -> Trigonometric Function/1
  ur/1 -> Demux/1
  Demux/1 -> [vr], Product/1
  Trigonometric Function/1 -> Product/2
  Product/1 -> Mux/1
  Demux/2 -> [wr], Mux/2
  Mux/1 -> u/1

== system Robot_Sim_bkp/Discriminator Block/discriminator1 ==
  value : Inport
  IN : Inport  Port=2
  Abs : Abs
  If : If  NumInputs=2  IfExpression=u1 < u2
  If Action Subsystem : Subsystem  TreatAsAtomicUnit=on
  If Action Subsystem1 : Subsystem  TreatAsAtomicUnit=on
  Merge : Merge
  OUT : Outport
  wires:
  IN/1 -> If Action Subsystem1/1(In1), Abs/1
  Abs/1 -> If/1
  If/1 -> If Action Subsystem/Action
  If/2 -> If Action Subsystem1/Action
  If Action Subsystem/1(Out1) -> Merge/1
  If Action Subsystem1/1(Out1) -> Merge/2
  Merge/1 -> OUT/1
  value/1 -> If/2

== system Robot_Sim_bkp/Discriminator Block/discriminator3 ==
  value : Inport
  IN : Inport  Port=2
  Abs : Abs
  If : If  NumInputs=2  IfExpression=u1 < u2
  If Action Subsystem : Subsystem  TreatAsAtomicUnit=on
  If Action Subsystem1 : Subsystem  TreatAsAtomicUnit=on
  Merge : Merge
  OUT : Outport
  wires:
  IN/1 -> If Action Subsystem1/1(In1), Abs/1
  Abs/1 -> If/1
  If/1 -> If Action Subsystem/Action
  If/2 -> If Action Subsystem1/Action
  If Action Subsystem/1(Out1) -> Merge/1
  If Action Subsystem1/1(Out1) -> Merge/2
  Merge/1 -> OUT/1
  value/1 -> If/2

== system Robot_Sim_bkp/discriminator5/If Action Subsystem ==
  Action Port : ActionPort  ActionType=then
  Constant : Constant  Value=0
  Out1 : Outport
  wires:
  Constant/1 -> Out1/1

== system Robot_Sim_bkp/discriminator5/If Action Subsystem1 ==
  In1 : Inport
  Action Port : ActionPort  ActionType=else
  Out1 : Outport
  wires:
  In1/1 -> Out1/1

== system Robot_Sim_bkp/Discriminator Block/discriminator1/If Action Subsystem ==
  Action Port : ActionPort  ActionType=then
  Constant : Constant  Value=0
  Out1 : Outport
  wires:
  Constant/1 -> Out1/1

== system Robot_Sim_bkp/Discriminator Block/discriminator1/If Action Subsystem1 ==
  In1 : Inport
  Action Port : ActionPort  ActionType=else
  Out1 : Outport
  wires:
  In1/1 -> Out1/1

== system Robot_Sim_bkp/Discriminator Block/discriminator3/If Action Subsystem ==
  Action Port : ActionPort  ActionType=then
  Constant : Constant  Value=0
  Out1 : Outport
  wires:
  Constant/1 -> Out1/1

== system Robot_Sim_bkp/Discriminator Block/discriminator3/If Action Subsystem1 ==
  In1 : Inport
  Action Port : ActionPort  ActionType=else
  Out1 : Outport
  wires:
  In1/1 -> Out1/1
